simulink model "Comparator"  (R2017a)
settings: Solver=VariableStepAuto  StartTime=0.0  StopTime=10.0  RelTol=1e-3
undefined symbols (not defined in the file or in its folder): High, T_maneuver
libraries: dspswit3 x2
settings Model: Creator=mtwal  LastModifiedBy=mtwal

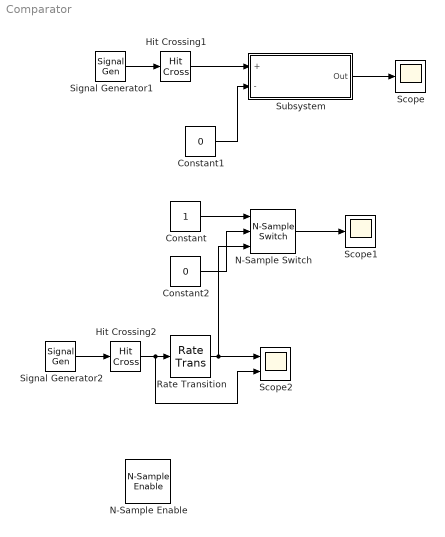
== system Comparator ==
  Constant : Constant
  Constant1 : Constant  Value=0
  Constant2 : Constant  Value=0
  Hit Crossing1 : HitCross  HitCrossingOffset=0.5  HitCrossingDirection=rising
  Hit Crossing2 : HitCross  HitCrossingOffset=0.5  HitCrossingDirection=rising
  N-Sample Enable : dspswit3/N-Sample Enable  N=8  ActiveLevel=High (1)  reset=on  TriggerType=Rising edge  Ts=1  DataType=Logical
      settings: SourceProductName=DSP System Toolbox  SourceProductBaseCode=DS
  N-Sample Switch : dspswit3/N-Sample Switch  N=1  reset=on  TriggerType=Rising edge  Ts=T_maneuver
      settings: SourceProductName=DSP System Toolbox  SourceProductBaseCode=DS
  Rate Transition : RateTransition  OutPortSampleTime=1
  Scope : Scope
  Scope1 : Scope
  Scope2 : Scope  NumInputPorts=2
  Signal Generator1 : SignalGenerator  Frequency=pi/3  Units=rad/sec
  Signal Generator2 : SignalGenerator  Frequency=pi/3  Units=rad/sec
  Subsystem : Subsystem
  wires:
  Constant1/1 -> Subsystem/2(-)
  Subsystem/1(Out) -> Scope/1
  Hit Crossing1/1 -> Subsystem/1(+)
  Signal Generator1/1 -> Hit Crossing1/1
  Constant/1 -> N-Sample Switch/1
  Constant2/1 -> N-Sample Switch/2
  N-Sample Switch/1 -> Scope1/1
  Signal Generator2/1 -> Hit Crossing2/1
  Hit Crossing2/1 -> Scope2/2, Rate Transition/1
  Rate Transition/1 -> N-Sample Switch/3, Scope2/1

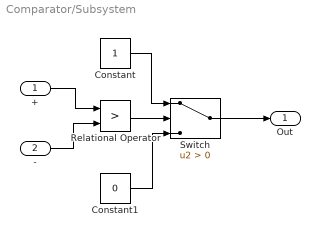
== system Comparator/Subsystem ==
  + : Inport
  - : Inport  Port=2
  Constant : Constant
  Constant1 : Constant  Value=0
  Relational Operator : RelationalOperator  Operator=>  OutDataTypeStr=boolean  RndMeth=Simplest
  Switch : Switch  Criteria=u2 > Threshold
  Out : Outport
  wires:
  +/1 -> Relational Operator/1
  -/1 -> Relational Operator/2
  Relational Operator/1 -> Switch/2
  Constant/1 -> Switch/1
  Constant1/1 -> Switch/3
  Switch/1 -> Out/1
